simulink model "ME655_Lect09_VL3_Simulink"  (R2023a)
settings: Solver=FixedStepAuto  StartTime=0.0  StopTime=60.0  FixedStep=.003  RelTol=1e-3
values from neighbouring files (symbols this model uses):
  A = [1 T; 0 1]    [MATLAB.m]    (also in ME655_Lect09_VL3_MATLAB.m)
  big_K = S_P * C / (S_H)    [MATLAB.m]    (also in ME655_Lect09_VL3_MATLAB.m)
  dt_active_control = 10    [MATLAB.m]    (also in ME655_Lect09_VL3_MATLAB.m)
  epsilon = 12    [MATLAB.m]    (also in ME655_Lect09_VL3_MATLAB.m)
  h = 2.5*N    (= 200)    [MATLAB.m]    (also in ME655_Lect09_VL3_MATLAB.m)
  lambda = .95    (= 0.95)    [MATLAB.m]    (also in ME655_Lect09_VL3_MATLAB.m)
  Lhip_pos0 = Lhip_pos(1)    [MATLAB.m]    (also in ME655_Lect09_VL3_MATLAB.m)
  Lhip_vel0 = Lhip_vel(1)    [MATLAB.m]    (also in ME655_Lect09_VL3_MATLAB.m)
  M = 6    [MATLAB.m]    (also in ME655_Lect09_VL3_MATLAB.m)
  N = 80    [MATLAB.m]    (also in ME655_Lect09_VL3_MATLAB.m)
  nu = .5    (= 0.5)    [MATLAB.m]    (also in ME655_Lect09_VL3_MATLAB.m)
  Q = G * G' * var(Lhip_a)    [MATLAB.m]    (also in ME655_Lect09_VL3_MATLAB.m)
  R = [var(phiP_dot_hat - Lhip_v) 0; 0 var(phiP_hat - Lhip_p)]    [MATLAB.m]    (also in ME655_Lect09_VL3_MATLAB.m)
  small_k = (-1) * big_K * phiH_avg' + phiP_avg'    [MATLAB.m]    (also in ME655_Lect09_VL3_MATLAB.m)
  t_start = 5.0    (= 5)    [MATLAB.m]    (also in ME655_Lect09_VL3_MATLAB.m)
  Tau_h_max = 30    [MATLAB.m]    (also in ME655_Lect09_VL3_MATLAB.m)
undefined symbols (not defined in the file or in its folder): Bh, g, IHC, IRC, Kh, LH, LR, mH, mR, theta_0, theta_d0
settings Model: Creator=Damiano  LastModifiedBy=hunte
settings SolverCC: AlgebraicLoopSolver=TrustRegion
settings DataIOCC: ReturnWorkspaceOutputs=off
settings DebuggingCC: UnconnectedInputMsg=warning  UnconnectedOutputMsg=warning  UnconnectedLineMsg=warning  ArithmeticOperatorsInVariantConditions=warning
settings ModelReferenceCC: EnableRefExpFcnMdlSchedulingChecks=on
settings SFSimCC: SimUseLocalCustomCode=off  CustomCodeUndefinedFunction=UseInterfaceOnly
settings RTWCC: RTWUseLocalCustomCode=off  DLArmComputeVersion=19.05
settings CodeAppCC: StateflowObjectComments=on

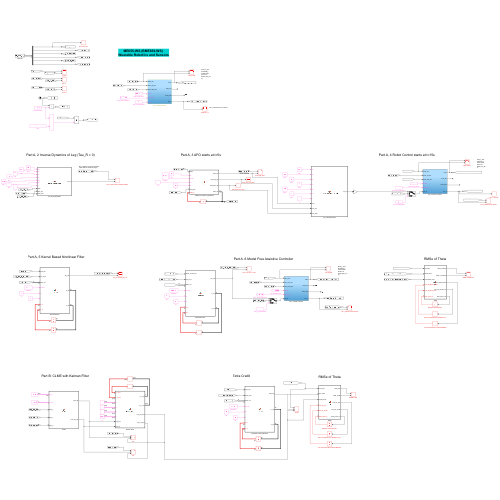
[thumbnail: Simulink's stored preview of the top-level diagram]
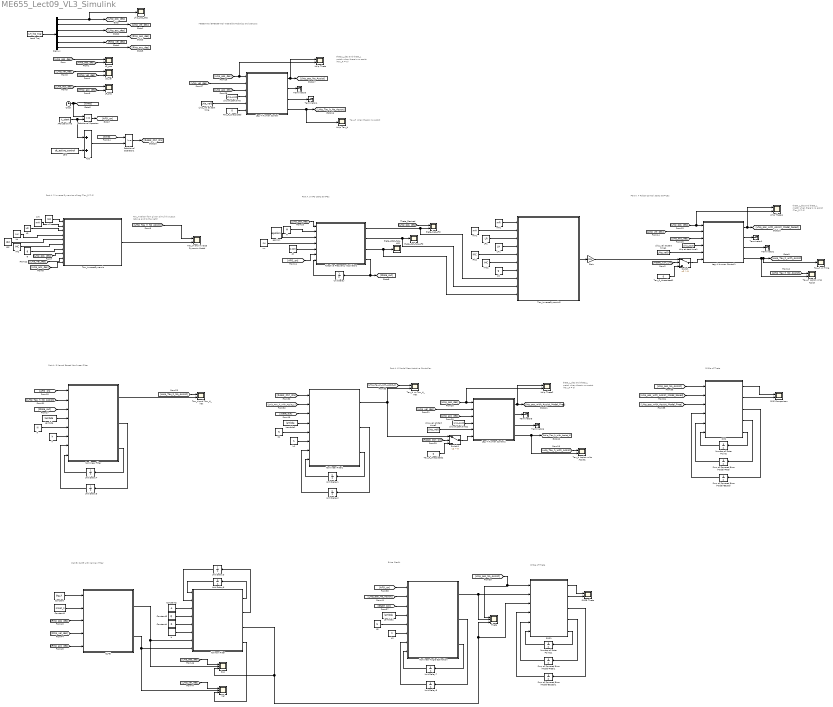
== system ME655_Lect09_VL3_Simulink ==
  note: Part A, 4 Robot Control starts at t=15s
  note: theta_L_des and theta_L match when there's no assist (Tau_R = 0)
  note: Part A, 5 Kernel Based Nonlinear Filter
  note: Part A, 3 AFO starts at t=5s
  note: theta_L_des and theta_L match when there's no assist (Tau_R = 0)
  note: ME655-WS (BME656-WS)
      | Wearable Robotics and Sensors
  note: Tau_H taken from given Simulink output (above and to the right)
  note: Part A, 2 Inverse Dynamics of Leg (Tau_R = 0)
  note: Tau_H when there's no assist
  note: theta_L_des and theta_L match when there's no assist (Tau_R = 0)
  note: Part A, 6 Model Free Assistive Controller
  note: RMSe of Theta
  note: Part B: CLME with Kalman Filter
  note: Extra Credit
  note: RMSe of Theta
  AFO start time : Constant  Value=t_start
  Adaptive Frequency Oscillators : MATLAB Function  TreatAsAtomicUnit=on
  Add : Sum
  CLME : MATLAB Function  TreatAsAtomicUnit=on
  Clock : Clock
  Constant : Constant  Value=big_K
  Constant1 : Constant  Value=small_k
  Constant2 : Constant  Value=A
  Constant3 : Constant  Value=Q
  Constant4 : Constant  Value=R
  Demux : Demux  Outputs=6
  Gain : Gain  Gain=0.5
  H : Constant  Value=eye(2)
  IHC : Constant  Value=IHC
  IHC1 : Constant  Value=IHC
  IRC : Constant  Value=IRC
  IRC1 : Constant  Value=IRC
  Kalman Filter : MATLAB Function  TreatAsAtomicUnit=on
  LH : Constant  Value=LH
  LH1 : Constant  Value=LH
  LHip Tau_H : Scope
  LHip Theta : Scope  NumInputPorts=2
  LHip Theta1 : Scope  NumInputPorts=2
  LHip Theta2 : Scope  NumInputPorts=2
  LR : Constant  Value=LR
  LR1 : Constant  Value=LR
  "LR_acc " : Scope  NumInputPorts=2
  LR_pos : Scope  NumInputPorts=2
  LR_vel : Scope  NumInputPorts=2
  Lambda : Constant  Value=lambda
  Lambda1 : Constant  Value=lambda
  Lambda2 : Constant  Value=lambda
  Leg + Human Control : Subsystem
  Leg + Human Control1 : Subsystem
  Leg + Human Control2 : Subsystem
  Lhip at start time : Constant  Value=Lhip_pos0
  Lhip at start time1 : Constant  Value=Lhip_pos0
  Lhip at start time2 : Constant  Value=Lhip_pos0
  Lhip_pos_des : Scope
  Lhip_vel at start time : Constant  Value=Lhip_vel0
  Lhip_vel at start time1 : Constant  Value=Lhip_vel0
  Lhip_vel at start time2 : Constant  Value=Lhip_vel0
  Load Traj : FromWorkspace  VariableName=LH_hip_traj
  M : Constant  Value=M
  N : Constant  Value=N
  N1 : Constant  Value=N
  N2 : Constant  Value=N
  Nonlinear Angle Estimation : MATLAB Function  TreatAsAtomicUnit=on
  Nonlinear Filter : MATLAB Function  TreatAsAtomicUnit=on
  Nonlinear Filter1 : MATLAB Function  TreatAsAtomicUnit=on
  Number of Data Points : UnitDelay  SampleTime=-1  HasFrameUpgradeWarning=on
  Number of Data Points1 : UnitDelay  SampleTime=-1  HasFrameUpgradeWarning=on
  Pos : Scope  NumInputPorts=3
  RMS : MATLAB Function  TreatAsAtomicUnit=on
  RMS Comparison : Scope  NumInputPorts=2
  RMS1 : MATLAB Function  TreatAsAtomicUnit=on
  RMSE Theta : Scope  NumInputPorts=2
  Relational Operator : RelationalOperator  OutDataTypeStr=boolean  RndMeth=Simplest  InputSameDT=off
  Relational Operator1 : RelationalOperator  OutDataTypeStr=boolean  RndMeth=Simplest  InputSameDT=off
  Sum of Squared Error (Model-Based) : UnitDelay  SampleTime=-1  HasFrameUpgradeWarning=on
  Sum of Squared Error (Model-Based)1 : UnitDelay  SampleTime=-1  HasFrameUpgradeWarning=on
  Sum of Squared Error (Model-Free) : UnitDelay  SampleTime=-1  HasFrameUpgradeWarning=on
  Sum of Squared Error (Model-Free)1 : UnitDelay  SampleTime=-1  HasFrameUpgradeWarning=on
  Switch : Switch  Criteria=u2 > Threshold  SaturateOnIntegerOverflow=off  InputSameDT=off
  Switch1 : Switch  Criteria=u2 > Threshold  SaturateOnIntegerOverflow=off  InputSameDT=off
  Tau_H Assist vs No Assist : Scope  NumInputPorts=2
  Tau_H Assist vs No Assist1 : Scope  NumInputPorts=2
  Tau_H and Inverse Dynamic Model : Scope  NumInputPorts=2
  Tau_H and Tau_H_hat : Scope  NumInputPorts=2
  Tau_H vs Tau_H_Hat : Scope  NumInputPorts=2
  Tau_InverseDynamic : MATLAB Function  TreatAsAtomicUnit=on
  Tau_InverseDynamic2 : MATLAB Function  TreatAsAtomicUnit=on
  Tau_R_Unassisted : Constant  Value=0
  Tau_R_Unassisted1 : Constant  Value=0
  Tau_R_Unassisted2 : Constant  Value=0
  Tau_h vs Time : Scope
  Terminator{1..6} (6 alike) : Terminator
  Theta : Scope  NumInputPorts=3
  Unit Delay : UnitDelay  InitialCondition=[0; 3*pi/2; pi/2; pi/2; pi/2; pi/2; pi/2; pi/2; 0; 0; 0; 0; 0; 0];  SampleTime=-1  HasFrameUpgradeWarning=on
  Unit Delay1 : UnitDelay  InitialCondition=zeros([N,1])  SampleTime=-1  HasFrameUpgradeWarning=on
  Unit Delay2 : UnitDelay  InitialCondition=ones([N,1])  SampleTime=-1  HasFrameUpgradeWarning=on
  Unit Delay3 : UnitDelay  InitialCondition=eye(2)  SampleTime=-1  HasFrameUpgradeWarning=on
  Unit Delay4 : UnitDelay  InitialCondition=zeros([N,1])  SampleTime=-1  HasFrameUpgradeWarning=on
  Unit Delay5 : UnitDelay  InitialCondition=ones([N,1])  SampleTime=-1  HasFrameUpgradeWarning=on
  Unit Delay6 : UnitDelay  InitialCondition=[0;0]  SampleTime=-1  HasFrameUpgradeWarning=on
  Unit Delay7 : UnitDelay  InitialCondition=zeros([N,1])  SampleTime=-1  HasFrameUpgradeWarning=on
  Unit Delay8 : UnitDelay  InitialCondition=ones([N,1])  SampleTime=-1  HasFrameUpgradeWarning=on
  Vel : Scope  NumInputPorts=3
  dt : Constant  Value=0.003
  epsilon : Constant  Value=epsilon
  g : Constant  Value=g
  g1 : Constant  Value=g
  h : Constant  Value=h
  h1 : Constant  Value=h
  h2 : Constant  Value=h
  mH : Constant  Value=mH
  mH1 : Constant  Value=mH
  mR : Constant  Value=mR
  mR1 : Constant  Value=mR
  nu : Constant  Value=nu
  theta_ddot_hat_AFO : Scope
  theta_dot_hat_AFO : Scope
  theta_hat_AFO : Scope  NumInputPorts=2
  zero : Constant  Value=dt_active_control
  wires:
  Tau_InverseDynamic2/1(Tau_tot) -> Gain/1
  IHC1/1 -> Tau_InverseDynamic2/6(IHC)
  IRC1/1 -> Tau_InverseDynamic2/5(IRC)
  g1/1 -> Tau_InverseDynamic2/7(g)
  LH1/1 -> Tau_InverseDynamic2/4(LH)
  LR1/1 -> Tau_InverseDynamic2/3(LR)
  mH1/1 -> Tau_InverseDynamic2/2(mH)
  mR1/1 -> Tau_InverseDynamic2/1(mR)
  [Lhip_pos_des] -> LHip Theta1/2, Leg + Human Control1/1(theta_des)
  Leg + Human Control1/4(Tau_h) -> Tau_h vs Time/1, [LHip_Tau_h_with_Assist], Tau_H Assist vs No Assist/2
  Leg + Human Control1/1(theta) -> [Lhip_pos_with_Assist_Model_based], LHip Theta1/1
  Lhip at start time1/1 -> Leg + Human Control1/4(theta0)
  [Lhip_vel_des] -> Leg + Human Control1/2(theta_dot_des)
  Leg + Human Control1/2(theta_dot) -> Terminator1/1
  Lhip_vel at start time1/1 -> Leg + Human Control1/5(theta0_dot)
  Leg + Human Control1/3(theta_ddot) -> Terminator2/1
  [Lhip_acc_des] -> Leg + Human Control1/3(theta_ddot_des)
  Gain/1 -> Switch/1
  Unit Delay4/1 -> Nonlinear Filter/8(w_in)
  h/1 -> Nonlinear Filter/6(h)
  Lambda/1 -> Nonlinear Filter/4(lambda)
  Nonlinear Filter/3(w_out) -> Unit Delay4/1
  Unit Delay5/1 -> Nonlinear Filter/7(P_in)
  N/1 -> Nonlinear Filter/5(N)
  [LHip_Tau_h_No_Assist] -> Nonlinear Filter/2(Tau_input)
  [State_out] -> Nonlinear Filter/3(State_out)
  LH/1 -> Tau_InverseDynamic/4(LH)
  Demux/2 -> [Lhip_vel_des]
  [Lhip_pos_des] -> theta_hat_AFO/1
  epsilon/1 -> Adaptive Frequency Oscillators/3(epsilon)
  Lhip at start time/1 -> Leg + Human Control/4(theta0)
  Demux/1 -> Lhip_pos_des/1, [Lhip_pos_des]
  Demux/6 -> [Rhip_acc_des]
  nu/1 -> Adaptive Frequency Oscillators/4(nu)
  Leg + Human Control/1(theta) -> LHip Theta/1, [Lhip_pos_No_Assist]
  Relational Operator/1 -> [AFO_on]
  LR/1 -> Tau_InverseDynamic/3(LR)
  [AFO_on] -> Adaptive Frequency Oscillators/6(AFO_ON)
  Adaptive Frequency Oscillators/3(theta_ddot_hat) -> Tau_InverseDynamic2/10(theta_ddot), theta_ddot_hat_AFO/1
  M/1 -> Adaptive Frequency Oscillators/2(M)
  Unit Delay/1 -> Adaptive Frequency Oscillators/7(state_in)
  Tau_InverseDynamic/1(Tau_tot) -> Tau_H and Inverse Dynamic Model/2
  Adaptive Frequency Oscillators/4(state_out) -> Unit Delay/1, [State_out]
  Demux/3 -> [Lhip_acc_des]
  Relational Operator1/1 -> [Robot_Ctrl_ON]
  [Lhip_acc_des] -> Tau_InverseDynamic/10(theta_ddot)
  [Lhip_acc_des] -> "LR_acc "/1
  Adaptive Frequency Oscillators/2(theta_dot_hat) -> Tau_InverseDynamic2/9(theta_dot), theta_dot_hat_AFO/1
  Leg + Human Control/2(theta_dot) -> Terminator3/1
  mH/1 -> Tau_InverseDynamic/2(mH)
  [Lhip_vel_des] -> LR_vel/1
  IHC/1 -> Tau_InverseDynamic/6(IHC)
  Leg + Human Control/4(Tau_h) -> LHip Tau_H/1, [LHip_Tau_h_No_Assist]
  g/1 -> Tau_InverseDynamic/7(g)
  Tau_R_Unassisted/1 -> Leg + Human Control/6(Tau_R)
  Adaptive Frequency Oscillators/1(theta_hat) -> Tau_InverseDynamic2/8(theta), theta_hat_AFO/2
  [Lhip_pos_des] -> Tau_InverseDynamic/8(theta)
  [LHip_Tau_h_No_Assist] -> Tau_H and Inverse Dynamic Model/1
  dt/1 -> Adaptive Frequency Oscillators/5(dt)
  zero/1 -> Add/2
  mR/1 -> Tau_InverseDynamic/1(mR)
  [Lhip_pos_des] -> Leg + Human Control/1(theta_des), LHip Theta/2
  [Lhip_acc_des] -> Leg + Human Control/3(theta_ddot_des)
  [Lhip_vel_des] -> Tau_InverseDynamic/9(theta_dot)
  [Lhip_pos_des] -> LR_pos/1
  Add/1 -> Relational Operator1/2
  IRC/1 -> Tau_InverseDynamic/5(IRC)
  [Rhip_vel_des] -> LR_vel/2
  Clock/1 -> Relational Operator/1, [time]
  Load Traj/1 -> Demux/1
  [Rhip_acc_des] -> "LR_acc "/2
  [Lhip_pos_des] -> Adaptive Frequency Oscillators/1(theta)
  [Lhip_vel_des] -> Leg + Human Control/2(theta_dot_des)
  Leg + Human Control/3(theta_ddot) -> Terminator4/1
  [time] -> Relational Operator1/1
  AFO start time/1 -> Add/1, Relational Operator/2
  Demux/4 -> [Rhip_pos_des]
  Demux/5 -> [Rhip_vel_des]
  Lhip_vel at start time/1 -> Leg + Human Control/5(theta0_dot)
  [Rhip_pos_des] -> LR_pos/2
  [LHip_Tau_h_No_Assist] -> Tau_H Assist vs No Assist/1
  Tau_R_Unassisted1/1 -> Switch/3
  [Robot_Ctrl_ON] -> Switch/2
  Switch/1 -> Leg + Human Control1/6(Tau_R)
  [AFO_on] -> Nonlinear Filter/1(AFO_ON)
  [LHip_Tau_h_No_Assist] -> Tau_H and Tau_H_hat/1
  [Robot_Ctrl_ON] -> Switch1/2
  Switch1/1 -> Leg + Human Control2/6(Tau_R)
  Nonlinear Filter/2(P_out) -> Unit Delay5/1
  Tau_R_Unassisted2/1 -> Switch1/3
  Lhip_vel at start time2/1 -> Leg + Human Control2/5(theta0_dot)
  [Lhip_pos_des] -> LHip Theta2/2, Leg + Human Control2/1(theta_des)
  Leg + Human Control2/3(theta_ddot) -> Terminator6/1
  Leg + Human Control2/1(theta) -> [Lhip_pos_with_Assist_Model_Free], LHip Theta2/1
  [Lhip_vel_des] -> Leg + Human Control2/2(theta_dot_des)
  Leg + Human Control2/4(Tau_h) -> [LHip_Tau_h_with_Assist_1], Tau_H Assist vs No Assist1/2
  [Lhip_acc_des] -> Leg + Human Control2/3(theta_ddot_des)
  Lhip at start time2/1 -> Leg + Human Control2/4(theta0)
  [LHip_Tau_h_with_Assist] -> Tau_H Assist vs No Assist1/1
  Leg + Human Control2/2(theta_dot) -> Terminator5/1
  Nonlinear Filter/1(Tau_hat) -> Tau_H and Tau_H_hat/2
  Nonlinear Filter1/2(P_out) -> Unit Delay2/1
  [Robot_Ctrl_ON] -> Nonlinear Filter1/1(Robot_Control_ON)
  [State_out] -> Nonlinear Filter1/3(State_out)
  [LHip_Tau_h_with_Assist_1] -> Nonlinear Filter1/2(Tau_input)
  N1/1 -> Nonlinear Filter1/5(N)
  Unit Delay2/1 -> Nonlinear Filter1/7(P_in)
  Nonlinear Filter1/3(w_out) -> Unit Delay1/1
  Lambda1/1 -> Nonlinear Filter1/4(lambda)
  h1/1 -> Nonlinear Filter1/6(h)
  Unit Delay1/1 -> Nonlinear Filter1/8(w_in)
  Nonlinear Filter1/1(Tau_hat) -> Tau_H vs Tau_H_Hat/2, Switch1/1
  [LHip_Tau_h_with_Assist_1] -> Tau_H vs Tau_H_Hat/1
  [Lhip_pos_with_Assist_Model_Free] -> RMS/3(Unmodeled_theta)
  [Lhip_pos_No_Assist] -> RMS/1(Act_theta)
  [Lhip_pos_with_Assist_Model_based] -> RMS/2(Model_theta)
  Number of Data Points/1 -> RMS/6(Data_points_in)
  Sum of Squared Error (Model-Free)/1 -> RMS/5("Sum_E2_Model_free ")
  Sum of Squared Error (Model-Based)/1 -> RMS/4("Sum_E2_Model_based ")
  RMS/1(RMS_modeled) -> RMS Comparison/1
  RMS/2(RMS_unmodeled) -> RMS Comparison/2
  RMS/5(Data_points_out) -> Number of Data Points/1
  RMS/4(Sum_E2_Model_free) -> Sum of Squared Error (Model-Free)/1
  RMS/3(Sum_E2_Model_based) -> Sum of Squared Error (Model-Based)/1
  CLME/2(phiP_dot_hat) -> Kalman Filter/8(Lhip_vel), Vel/2
  Unit Delay3/1 -> Kalman Filter/2(P_k_prev)
  [Rhip_pos_des] -> CLME/3(Rhip_p)
  [Rhip_acc_des] -> CLME/5(Rhip_a)
  CLME/1(phiP_hat) -> Kalman Filter/7(Lhip_pos), Pos/2
  [Rhip_vel_des] -> CLME/4(Rhip_v)
  Kalman Filter/2(P_k_next) -> Unit Delay3/1
  Unit Delay6/1 -> Kalman Filter/1(x_k_prev)
  Kalman Filter/1(x_k_next) -> Unit Delay6/1
  H/1 -> Kalman Filter/6(H)
  Kalman Filter/4(Lhip_vel_des) -> Vel/3
  [Lhip_pos_des] -> Pos/1
  [Lhip_vel_des] -> Vel/1
  Constant1/1 -> CLME/2(small_k)
  Constant/1 -> CLME/1(big_K)
  Constant2/1 -> Kalman Filter/3(A)
  Constant3/1 -> Kalman Filter/4(Q)
  Constant4/1 -> Kalman Filter/5(R)
  N2/1 -> Nonlinear Angle Estimation/5(N)
  h2/1 -> Nonlinear Angle Estimation/6(h)
  Nonlinear Angle Estimation/2(P_out) -> Unit Delay8/1
  Nonlinear Angle Estimation/3(w_out) -> Unit Delay7/1
  Lambda2/1 -> Nonlinear Angle Estimation/4(lambda)
  Unit Delay8/1 -> Nonlinear Angle Estimation/7(P_in)
  [State_out] -> Nonlinear Angle Estimation/3(State_out)
  [AFO_on] -> Nonlinear Angle Estimation/1(AFO_ON)
  Unit Delay7/1 -> Nonlinear Angle Estimation/8(w_in)
  [Lhip_pos_No_Assist] -> Nonlinear Angle Estimation/2(theta_input)
  RMS1/3(Sum_E2_NLF) -> Sum of Squared Error (Model-Based)1/1
  RMS1/4(Sum_E2_CLME) -> Sum of Squared Error (Model-Free)1/1
  Sum of Squared Error (Model-Free)1/1 -> RMS1/5(Sum_E_CLME)
  RMS1/5(Data_points_out) -> Number of Data Points1/1
  Number of Data Points1/1 -> RMS1/6(Data_points_in)
  Kalman Filter/3(Lhip_pos_des) -> Pos/3, Theta/3, RMS1/3(CLME_theta)
  [Lhip_pos_No_Assist] -> Theta/1, RMS1/1(Act_theta)
  Nonlinear Angle Estimation/1(theta_hat) -> RMS1/2(NLF_theta), Theta/2
  Sum of Squared Error (Model-Based)1/1 -> RMS1/4(Sum_E_NLF)
  RMS1/1(RMS_NLF) -> RMSE Theta/1
  RMS1/2(RMS_CLME) -> RMSE Theta/2

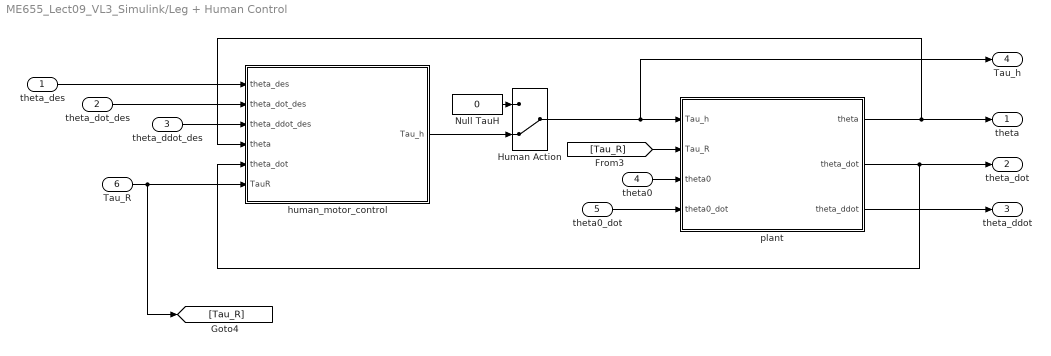
== system ME655_Lect09_VL3_Simulink/Leg + Human Control ==
  theta_des : Inport
  theta_dot_des : Inport  Port=2
  theta_ddot_des : Inport  Port=3
  theta0 : Inport  Port=4
  theta0_dot : Inport  Port=5
  Tau_R : Inport  Port=6
  Human Action : ManualSwitch  CurrentSetting=0
  Null TauH : Constant  Value=0
  human_motor_control : Subsystem
  plant : Subsystem
  theta : Outport  PortDimensions=[1,1]  VectorParamsAs1DForOutWhenUnconnected=off
  theta_dot : Outport  Port=2  PortDimensions=[1,1]  VectorParamsAs1DForOutWhenUnconnected=off
  theta_ddot : Outport  Port=3  PortDimensions=[1,1]  VectorParamsAs1DForOutWhenUnconnected=off
  Tau_h : Outport  Port=4  PortDimensions=[1,1]  VectorParamsAs1DForOutWhenUnconnected=off
  wires:
  theta_des/1 -> human_motor_control/1(theta_des)
  theta_dot_des/1 -> human_motor_control/2(theta_dot_des)
  theta0/1 -> plant/3(theta0)
  theta0_dot/1 -> plant/4(theta0_dot)
  [Tau_R] -> plant/2(Tau_R)
  plant/1(theta) -> theta/1, human_motor_control/4(theta)
  plant/2(theta_dot) -> human_motor_control/5(theta_dot), theta_dot/1
  plant/3(theta_ddot) -> theta_ddot/1
  theta_ddot_des/1 -> human_motor_control/3(theta_ddot_des)
  human_motor_control/1(Tau_h) -> Human Action/2
  Human Action/1 -> Tau_h/1, plant/1(Tau_h)
  Null TauH/1 -> Human Action/1
  Tau_R/1 -> [Tau_R], human_motor_control/6(TauR)

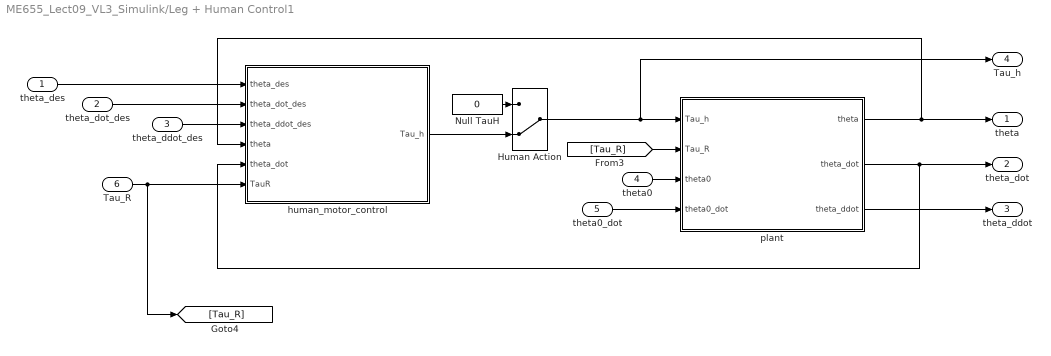
== system ME655_Lect09_VL3_Simulink/Leg + Human Control1 ==
  theta_des : Inport
  theta_dot_des : Inport  Port=2
  theta_ddot_des : Inport  Port=3
  theta0 : Inport  Port=4
  theta0_dot : Inport  Port=5
  Tau_R : Inport  Port=6
  Human Action : ManualSwitch  CurrentSetting=0
  Null TauH : Constant  Value=0
  human_motor_control : Subsystem
  plant : Subsystem
  theta : Outport  PortDimensions=[1,1]  VectorParamsAs1DForOutWhenUnconnected=off
  theta_dot : Outport  Port=2  PortDimensions=[1,1]  VectorParamsAs1DForOutWhenUnconnected=off
  theta_ddot : Outport  Port=3  PortDimensions=[1,1]  VectorParamsAs1DForOutWhenUnconnected=off
  Tau_h : Outport  Port=4  PortDimensions=[1,1]  VectorParamsAs1DForOutWhenUnconnected=off
  wires:
  Tau_R/1 -> human_motor_control/6(TauR), [Tau_R]
  Null TauH/1 -> Human Action/1
  Human Action/1 -> plant/1(Tau_h), Tau_h/1
  human_motor_control/1(Tau_h) -> Human Action/2
  theta_ddot_des/1 -> human_motor_control/3(theta_ddot_des)
  plant/3(theta_ddot) -> theta_ddot/1
  plant/2(theta_dot) -> theta_dot/1, human_motor_control/5(theta_dot)
  plant/1(theta) -> human_motor_control/4(theta), theta/1
  [Tau_R] -> plant/2(Tau_R)
  theta0_dot/1 -> plant/4(theta0_dot)
  theta0/1 -> plant/3(theta0)
  theta_dot_des/1 -> human_motor_control/2(theta_dot_des)
  theta_des/1 -> human_motor_control/1(theta_des)

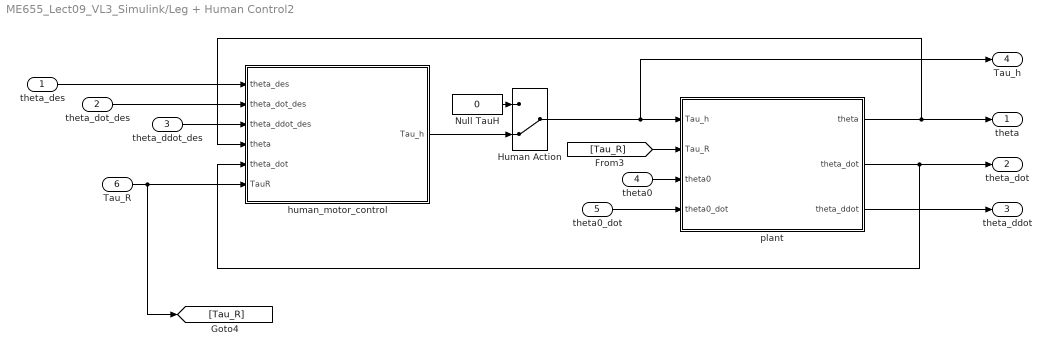
== system ME655_Lect09_VL3_Simulink/Leg + Human Control2 ==
  theta_des : Inport
  theta_dot_des : Inport  Port=2
  theta_ddot_des : Inport  Port=3
  theta0 : Inport  Port=4
  theta0_dot : Inport  Port=5
  Tau_R : Inport  Port=6
  Human Action : ManualSwitch  CurrentSetting=0
  Null TauH : Constant  Value=0
  human_motor_control : Subsystem
  plant : Subsystem
  theta : Outport  PortDimensions=[1,1]  VectorParamsAs1DForOutWhenUnconnected=off
  theta_dot : Outport  Port=2  PortDimensions=[1,1]  VectorParamsAs1DForOutWhenUnconnected=off
  theta_ddot : Outport  Port=3  PortDimensions=[1,1]  VectorParamsAs1DForOutWhenUnconnected=off
  Tau_h : Outport  Port=4  PortDimensions=[1,1]  VectorParamsAs1DForOutWhenUnconnected=off
  wires:
  Tau_R/1 -> human_motor_control/6(TauR), [Tau_R]
  Null TauH/1 -> Human Action/1
  Human Action/1 -> plant/1(Tau_h), Tau_h/1
  human_motor_control/1(Tau_h) -> Human Action/2
  theta_ddot_des/1 -> human_motor_control/3(theta_ddot_des)
  plant/3(theta_ddot) -> theta_ddot/1
  plant/2(theta_dot) -> theta_dot/1, human_motor_control/5(theta_dot)
  plant/1(theta) -> human_motor_control/4(theta), theta/1
  [Tau_R] -> plant/2(Tau_R)
  theta0_dot/1 -> plant/4(theta0_dot)
  theta0/1 -> plant/3(theta0)
  theta_dot_des/1 -> human_motor_control/2(theta_dot_des)
  theta_des/1 -> human_motor_control/1(theta_des)

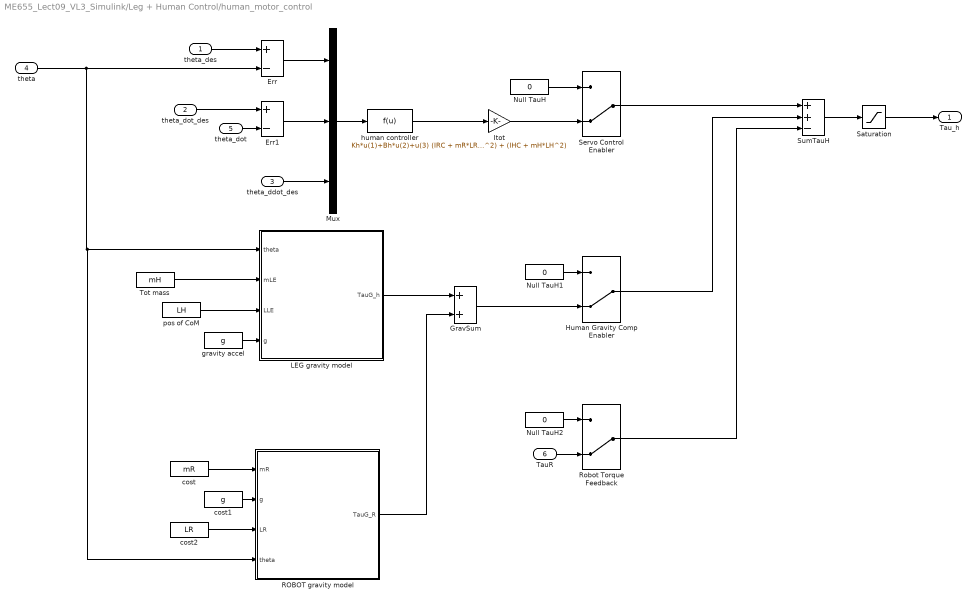
== system ME655_Lect09_VL3_Simulink/Leg + Human Control/human_motor_control ==
  theta_des : Inport
  theta_dot_des : Inport  Port=2
  theta_ddot_des : Inport  Port=3
  theta : Inport  Port=4
  theta_dot : Inport  Port=5
  TauR : Inport  Port=6
  Err : Sum  Inputs=+-
  Err1 : Sum  Inputs=+-
  GravSum : Sum
  Human Gravity Comp Enabler : ManualSwitch  CurrentSetting=0
  Itot : Gain  Gain=(IRC + mR*LR^2) + (IHC + mH*LH^2)
  LEG gravity model : MATLAB Function  TreatAsAtomicUnit=on
  Mux : Mux  Inputs=3
  Null TauH : Constant  Value=0
  Null TauH1 : Constant  Value=0
  Null TauH2 : Constant  Value=0
  ROBOT gravity model : MATLAB Function  TreatAsAtomicUnit=on
  Robot Torque Feedback : ManualSwitch  CurrentSetting=0
  Saturation : Saturate  UpperLimit=Tau_h_max  LowerLimit=-Tau_h_max
  Servo Control Enabler : ManualSwitch  CurrentSetting=0
  SumTauH : Sum  Inputs=++-
  Tot mass : Constant  Value=mH
  cost : Constant  Value=mR
  cost1 : Constant  Value=g
  cost2 : Constant  Value=LR
  gravity accel : Constant  Value=g
  human controller : Fcn  Expr=Kh*u(1)+Bh*u(2)+u(3)
  pos of CoM : Constant  Value=LH
  Tau_h : Outport  PortDimensions=[1,1]  VectorParamsAs1DForOutWhenUnconnected=off
  wires:
  theta_des/1 -> Err/1
  theta_dot_des/1 -> Err1/1
  theta_dot/1 -> Err1/2
  Err/1 -> Mux/1
  Err1/1 -> Mux/2
  Mux/1 -> human controller/1
  theta_ddot_des/1 -> Mux/3
  gravity accel/1 -> LEG gravity model/4(g)
  Tot mass/1 -> LEG gravity model/2(mLE)
  pos of CoM/1 -> LEG gravity model/3(LLE)
  Null TauH/1 -> Servo Control Enabler/1
  Null TauH1/1 -> Human Gravity Comp Enabler/1
  Human Gravity Comp Enabler/1 -> SumTauH/2
  SumTauH/1 -> Saturation/1
  human controller/1 -> Itot/1
  Servo Control Enabler/1 -> SumTauH/1
  Saturation/1 -> Tau_h/1
  Itot/1 -> Servo Control Enabler/2
  Null TauH2/1 -> Robot Torque Feedback/1
  TauR/1 -> Robot Torque Feedback/2
  Robot Torque Feedback/1 -> SumTauH/3
  theta/1 -> ROBOT gravity model/4(theta), LEG gravity model/1(theta), Err/2
  ROBOT gravity model/1(TauG_R) -> GravSum/2
  cost2/1 -> ROBOT gravity model/3(LR)
  cost/1 -> ROBOT gravity model/1(mR)
  cost1/1 -> ROBOT gravity model/2(g)
  LEG gravity model/1(TauG_h) -> GravSum/1
  GravSum/1 -> Human Gravity Comp Enabler/2

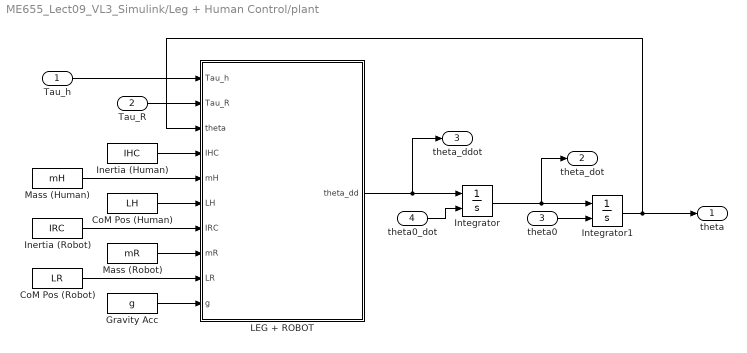
== system ME655_Lect09_VL3_Simulink/Leg + Human Control/plant ==
  Tau_h : Inport
  Tau_R : Inport  Port=2
  theta0 : Inport  Port=3
  theta0_dot : Inport  Port=4
  CoM Pos (Human) : Constant  Value=LH
  CoM Pos (Robot) : Constant  Value=LR
  Gravity Acc : Constant  Value=g
  Inertia (Human) : Constant  Value=IHC
  Inertia (Robot) : Constant  Value=IRC
  Integrator : Integrator  InitialConditionSource=external  InitialCondition=theta_d0
  Integrator1 : Integrator  InitialConditionSource=external  InitialCondition=theta_0
  LEG + ROBOT : MATLAB Function  TreatAsAtomicUnit=on
  Mass (Human) : Constant  Value=mH
  Mass (Robot) : Constant  Value=mR
  theta : Outport  PortDimensions=[1,1]  VectorParamsAs1DForOutWhenUnconnected=off
  theta_dot : Outport  Port=2  PortDimensions=[1,1]  VectorParamsAs1DForOutWhenUnconnected=off
  theta_ddot : Outport  Port=3  PortDimensions=[1,1]  VectorParamsAs1DForOutWhenUnconnected=off
  wires:
  Tau_h/1 -> LEG + ROBOT/1(Tau_h)
  Tau_R/1 -> LEG + ROBOT/2(Tau_R)
  LEG + ROBOT/1(theta_dd) -> theta_ddot/1, Integrator/1
  Integrator/1 -> theta_dot/1, Integrator1/1
  theta0_dot/1 -> Integrator/2
  theta0/1 -> Integrator1/2
  Integrator1/1 -> LEG + ROBOT/3(theta), theta/1
  Inertia (Human)/1 -> LEG + ROBOT/4(IHC)
  Mass (Human)/1 -> LEG + ROBOT/5(mH)
  CoM Pos (Human)/1 -> LEG + ROBOT/6(LH)
  Gravity Acc/1 -> LEG + ROBOT/10(g)
  Mass (Robot)/1 -> LEG + ROBOT/8(mR)
  CoM Pos (Robot)/1 -> LEG + ROBOT/9(LR)
  Inertia (Robot)/1 -> LEG + ROBOT/7(IRC)

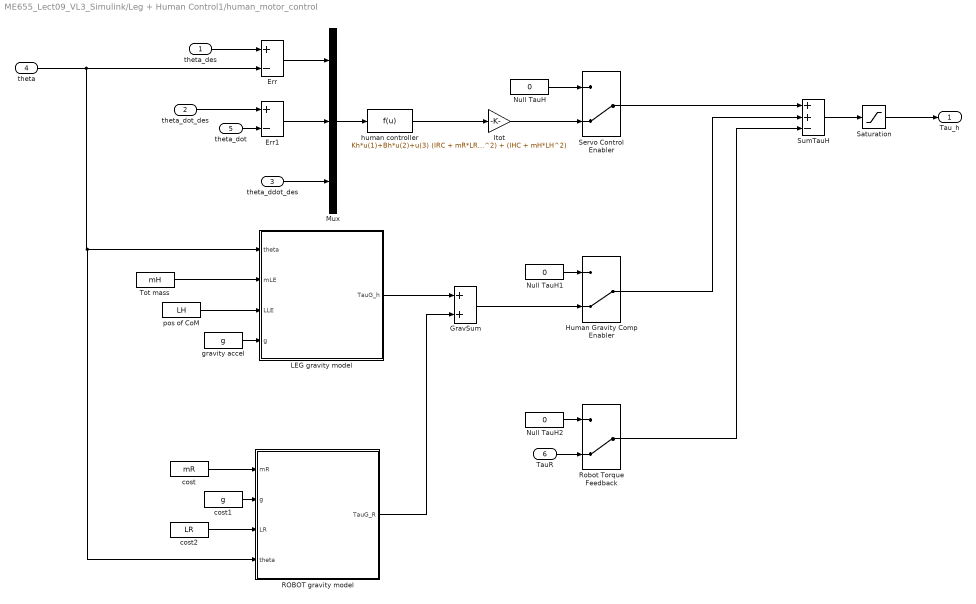
== system ME655_Lect09_VL3_Simulink/Leg + Human Control1/human_motor_control ==
  theta_des : Inport
  theta_dot_des : Inport  Port=2
  theta_ddot_des : Inport  Port=3
  theta : Inport  Port=4
  theta_dot : Inport  Port=5
  TauR : Inport  Port=6
  Err : Sum  Inputs=+-
  Err1 : Sum  Inputs=+-
  GravSum : Sum
  Human Gravity Comp Enabler : ManualSwitch  CurrentSetting=0
  Itot : Gain  Gain=(IRC + mR*LR^2) + (IHC + mH*LH^2)
  LEG gravity model : MATLAB Function  TreatAsAtomicUnit=on
  Mux : Mux  Inputs=3
  Null TauH : Constant  Value=0
  Null TauH1 : Constant  Value=0
  Null TauH2 : Constant  Value=0
  ROBOT gravity model : MATLAB Function  TreatAsAtomicUnit=on
  Robot Torque Feedback : ManualSwitch  CurrentSetting=0
  Saturation : Saturate  UpperLimit=Tau_h_max  LowerLimit=-Tau_h_max
  Servo Control Enabler : ManualSwitch  CurrentSetting=0
  SumTauH : Sum  Inputs=++-
  Tot mass : Constant  Value=mH
  cost : Constant  Value=mR
  cost1 : Constant  Value=g
  cost2 : Constant  Value=LR
  gravity accel : Constant  Value=g
  human controller : Fcn  Expr=Kh*u(1)+Bh*u(2)+u(3)
  pos of CoM : Constant  Value=LH
  Tau_h : Outport  PortDimensions=[1,1]  VectorParamsAs1DForOutWhenUnconnected=off
  wires:
  GravSum/1 -> Human Gravity Comp Enabler/2
  LEG gravity model/1(TauG_h) -> GravSum/1
  cost1/1 -> ROBOT gravity model/2(g)
  cost/1 -> ROBOT gravity model/1(mR)
  cost2/1 -> ROBOT gravity model/3(LR)
  ROBOT gravity model/1(TauG_R) -> GravSum/2
  theta/1 -> Err/2, LEG gravity model/1(theta), ROBOT gravity model/4(theta)
  Robot Torque Feedback/1 -> SumTauH/3
  TauR/1 -> Robot Torque Feedback/2
  Null TauH2/1 -> Robot Torque Feedback/1
  Itot/1 -> Servo Control Enabler/2
  Saturation/1 -> Tau_h/1
  Servo Control Enabler/1 -> SumTauH/1
  human controller/1 -> Itot/1
  SumTauH/1 -> Saturation/1
  Human Gravity Comp Enabler/1 -> SumTauH/2
  Null TauH1/1 -> Human Gravity Comp Enabler/1
  Null TauH/1 -> Servo Control Enabler/1
  pos of CoM/1 -> LEG gravity model/3(LLE)
  Tot mass/1 -> LEG gravity model/2(mLE)
  gravity accel/1 -> LEG gravity model/4(g)
  theta_ddot_des/1 -> Mux/3
  Mux/1 -> human controller/1
  Err1/1 -> Mux/2
  Err/1 -> Mux/1
  theta_dot/1 -> Err1/2
  theta_dot_des/1 -> Err1/1
  theta_des/1 -> Err/1

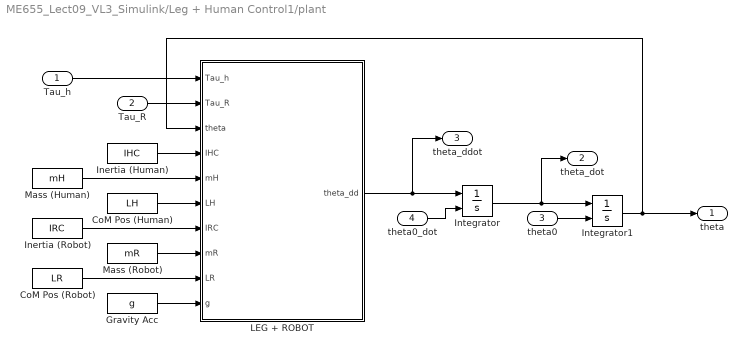
== system ME655_Lect09_VL3_Simulink/Leg + Human Control1/plant ==
  Tau_h : Inport
  Tau_R : Inport  Port=2
  theta0 : Inport  Port=3
  theta0_dot : Inport  Port=4
  CoM Pos (Human) : Constant  Value=LH
  CoM Pos (Robot) : Constant  Value=LR
  Gravity Acc : Constant  Value=g
  Inertia (Human) : Constant  Value=IHC
  Inertia (Robot) : Constant  Value=IRC
  Integrator : Integrator  InitialConditionSource=external  InitialCondition=theta_d0
  Integrator1 : Integrator  InitialConditionSource=external  InitialCondition=theta_0
  LEG + ROBOT : MATLAB Function  TreatAsAtomicUnit=on
  Mass (Human) : Constant  Value=mH
  Mass (Robot) : Constant  Value=mR
  theta : Outport  PortDimensions=[1,1]  VectorParamsAs1DForOutWhenUnconnected=off
  theta_dot : Outport  Port=2  PortDimensions=[1,1]  VectorParamsAs1DForOutWhenUnconnected=off
  theta_ddot : Outport  Port=3  PortDimensions=[1,1]  VectorParamsAs1DForOutWhenUnconnected=off
  wires:
  Inertia (Robot)/1 -> LEG + ROBOT/7(IRC)
  CoM Pos (Robot)/1 -> LEG + ROBOT/9(LR)
  Mass (Robot)/1 -> LEG + ROBOT/8(mR)
  Gravity Acc/1 -> LEG + ROBOT/10(g)
  CoM Pos (Human)/1 -> LEG + ROBOT/6(LH)
  Mass (Human)/1 -> LEG + ROBOT/5(mH)
  Inertia (Human)/1 -> LEG + ROBOT/4(IHC)
  Integrator1/1 -> theta/1, LEG + ROBOT/3(theta)
  theta0/1 -> Integrator1/2
  theta0_dot/1 -> Integrator/2
  Integrator/1 -> Integrator1/1, theta_dot/1
  LEG + ROBOT/1(theta_dd) -> Integrator/1, theta_ddot/1
  Tau_R/1 -> LEG + ROBOT/2(Tau_R)
  Tau_h/1 -> LEG + ROBOT/1(Tau_h)

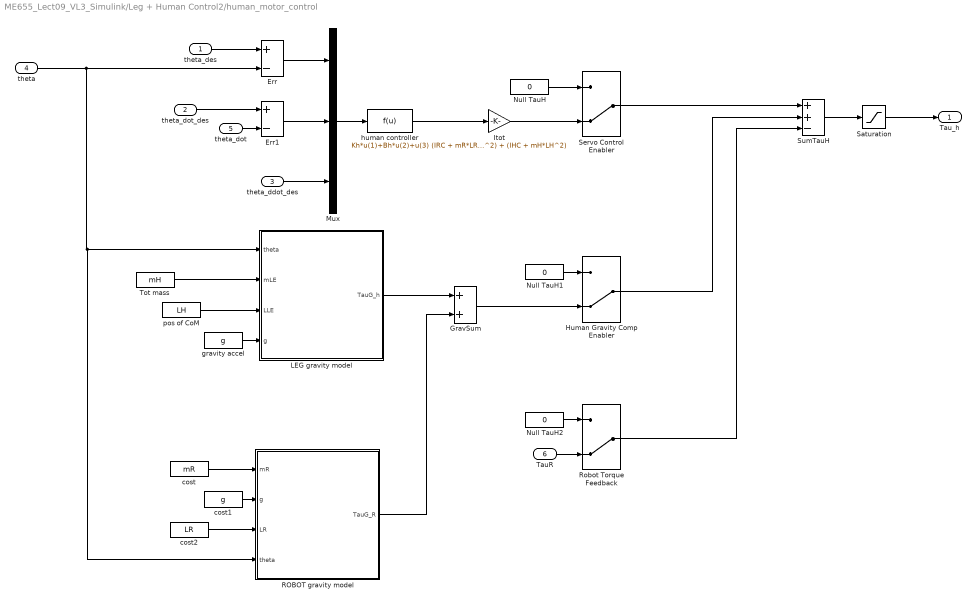
== system ME655_Lect09_VL3_Simulink/Leg + Human Control2/human_motor_control ==
  theta_des : Inport
  theta_dot_des : Inport  Port=2
  theta_ddot_des : Inport  Port=3
  theta : Inport  Port=4
  theta_dot : Inport  Port=5
  TauR : Inport  Port=6
  Err : Sum  Inputs=+-
  Err1 : Sum  Inputs=+-
  GravSum : Sum
  Human Gravity Comp Enabler : ManualSwitch  CurrentSetting=0
  Itot : Gain  Gain=(IRC + mR*LR^2) + (IHC + mH*LH^2)
  LEG gravity model : MATLAB Function  TreatAsAtomicUnit=on
  Mux : Mux  Inputs=3
  Null TauH : Constant  Value=0
  Null TauH1 : Constant  Value=0
  Null TauH2 : Constant  Value=0
  ROBOT gravity model : MATLAB Function  TreatAsAtomicUnit=on
  Robot Torque Feedback : ManualSwitch  CurrentSetting=0
  Saturation : Saturate  UpperLimit=Tau_h_max  LowerLimit=-Tau_h_max
  Servo Control Enabler : ManualSwitch  CurrentSetting=0
  SumTauH : Sum  Inputs=++-
  Tot mass : Constant  Value=mH
  cost : Constant  Value=mR
  cost1 : Constant  Value=g
  cost2 : Constant  Value=LR
  gravity accel : Constant  Value=g
  human controller : Fcn  Expr=Kh*u(1)+Bh*u(2)+u(3)
  pos of CoM : Constant  Value=LH
  Tau_h : Outport  PortDimensions=[1,1]  VectorParamsAs1DForOutWhenUnconnected=off
  wires:
  GravSum/1 -> Human Gravity Comp Enabler/2
  LEG gravity model/1(TauG_h) -> GravSum/1
  cost1/1 -> ROBOT gravity model/2(g)
  cost/1 -> ROBOT gravity model/1(mR)
  cost2/1 -> ROBOT gravity model/3(LR)
  ROBOT gravity model/1(TauG_R) -> GravSum/2
  theta/1 -> Err/2, LEG gravity model/1(theta), ROBOT gravity model/4(theta)
  Robot Torque Feedback/1 -> SumTauH/3
  TauR/1 -> Robot Torque Feedback/2
  Null TauH2/1 -> Robot Torque Feedback/1
  Itot/1 -> Servo Control Enabler/2
  Saturation/1 -> Tau_h/1
  Servo Control Enabler/1 -> SumTauH/1
  human controller/1 -> Itot/1
  SumTauH/1 -> Saturation/1
  Human Gravity Comp Enabler/1 -> SumTauH/2
  Null TauH1/1 -> Human Gravity Comp Enabler/1
  Null TauH/1 -> Servo Control Enabler/1
  pos of CoM/1 -> LEG gravity model/3(LLE)
  Tot mass/1 -> LEG gravity model/2(mLE)
  gravity accel/1 -> LEG gravity model/4(g)
  theta_ddot_des/1 -> Mux/3
  Mux/1 -> human controller/1
  Err1/1 -> Mux/2
  Err/1 -> Mux/1
  theta_dot/1 -> Err1/2
  theta_dot_des/1 -> Err1/1
  theta_des/1 -> Err/1

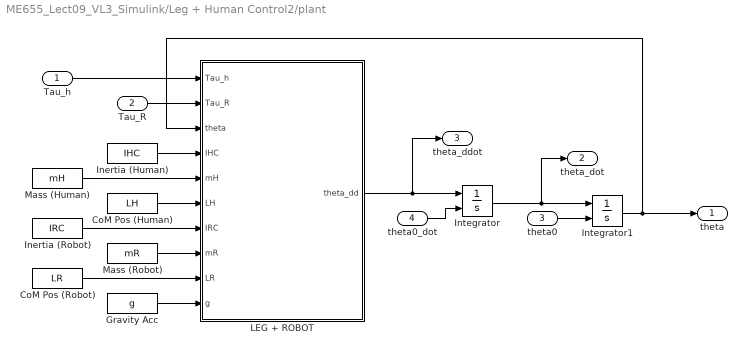
== system ME655_Lect09_VL3_Simulink/Leg + Human Control2/plant ==
  Tau_h : Inport
  Tau_R : Inport  Port=2
  theta0 : Inport  Port=3
  theta0_dot : Inport  Port=4
  CoM Pos (Human) : Constant  Value=LH
  CoM Pos (Robot) : Constant  Value=LR
  Gravity Acc : Constant  Value=g
  Inertia (Human) : Constant  Value=IHC
  Inertia (Robot) : Constant  Value=IRC
  Integrator : Integrator  InitialConditionSource=external  InitialCondition=theta_d0
  Integrator1 : Integrator  InitialConditionSource=external  InitialCondition=theta_0
  LEG + ROBOT : MATLAB Function  TreatAsAtomicUnit=on
  Mass (Human) : Constant  Value=mH
  Mass (Robot) : Constant  Value=mR
  theta : Outport  PortDimensions=[1,1]  VectorParamsAs1DForOutWhenUnconnected=off
  theta_dot : Outport  Port=2  PortDimensions=[1,1]  VectorParamsAs1DForOutWhenUnconnected=off
  theta_ddot : Outport  Port=3  PortDimensions=[1,1]  VectorParamsAs1DForOutWhenUnconnected=off
  wires:
  Inertia (Robot)/1 -> LEG + ROBOT/7(IRC)
  CoM Pos (Robot)/1 -> LEG + ROBOT/9(LR)
  Mass (Robot)/1 -> LEG + ROBOT/8(mR)
  Gravity Acc/1 -> LEG + ROBOT/10(g)
  CoM Pos (Human)/1 -> LEG + ROBOT/6(LH)
  Mass (Human)/1 -> LEG + ROBOT/5(mH)
  Inertia (Human)/1 -> LEG + ROBOT/4(IHC)
  Integrator1/1 -> theta/1, LEG + ROBOT/3(theta)
  theta0/1 -> Integrator1/2
  theta0_dot/1 -> Integrator/2
  Integrator/1 -> Integrator1/1, theta_dot/1
  LEG + ROBOT/1(theta_dd) -> Integrator/1, theta_ddot/1
  Tau_R/1 -> LEG + ROBOT/2(Tau_R)
  Tau_h/1 -> LEG + ROBOT/1(Tau_h)

== matlab function ME655_Lect09_VL3_Simulink/Nonlinear Filter ==
  data: AFO_ON input; Tau_hat output; Tau_input input; State_out input; lambda input; N input; h input; P_in input; w_in input; P_out output; w_out output
function [Tau_hat, P_out, w_out]= nonlin_filter(AFO_ON, Tau_input, State_out, lambda, N, h, P_in, w_in)

phi = State_out(3);

Tau_hat = 0;
P_out = P_in;
w_out = w_in;

if AFO_ON == 1

    Num = 0;
    Den = 0;
    err = zeros(N, 1);
    for i = 1:N
        psi = exp(h*(cos(phi - 2*pi*(i)/N)- 1));
        err(i) = Tau_input - w_in(i);
        P_out(i) = (1/lambda)*(P_in(i) - ((P_in(i)^2) / ((lambda/psi) + P_in(i))));    
        w_out(i) = w_in(i) + psi* P_out(i) * err(i);
        Num = Num + psi*w_in(i);
        Den = Den + psi;
    end

    Tau_hat = Num/Den;

end

== matlab function ME655_Lect09_VL3_Simulink/Leg + Human Control2/human_motor_control/LEG gravity model ==
  data: theta input; mLE input; LLE input; TauG_h output; g input
function TauG_h   = HumanLegGravModel(theta,mLE,LLE,g)
% human gravity compensation term
TauG_h=mLE*g*LLE*sin(theta);

end

== matlab function ME655_Lect09_VL3_Simulink/Leg + Human Control/human_motor_control/LEG gravity model ==
  data: theta input; mLE input; LLE input; TauG_h output; g input
function TauG_h   = HumanLegGravModel(theta,mLE,LLE,g)
% human gravity compensation term
TauG_h=mLE*g*LLE*sin(theta);

end

== matlab function ME655_Lect09_VL3_Simulink/Leg + Human Control2/human_motor_control/ROBOT gravity model ==
  data: mR input; g input; LR input; theta input; TauG_R output
function TauG_R  = RobotGravModel(mR,g,LR,theta)

TauG_R=mR*g*LR*sin(theta);
% TauG_h=mLE*g*LLE*sin(theta);

end

== matlab function ME655_Lect09_VL3_Simulink/Leg + Human Control2/plant/LEG + ROBOT ==
  data: Tau_h input; Tau_R input; theta input; theta_dd output; IHC input; mH input; LH input; IRC input; mR input; LR input; g input
function theta_dd   = LegRobotModel(Tau_h,Tau_R,theta,IHC,mH,LH,IRC,mR,LR,g)

theta_dd = 1/((IRC + mR*LR^2)+(IHC + mH*LH^2)) * (Tau_h-mH*g*LH*sin(theta) + Tau_R-mR*g*LR*sin(theta));

end

== matlab function ME655_Lect09_VL3_Simulink/Leg + Human Control/human_motor_control/ROBOT gravity model ==
  data: mR input; g input; LR input; theta input; TauG_R output
function TauG_R  = RobotGravModel(mR,g,LR,theta)

TauG_R=mR*g*LR*sin(theta);
% TauG_h=mLE*g*LLE*sin(theta);

end

== matlab function ME655_Lect09_VL3_Simulink/Nonlinear Filter1 ==
  data: Robot_Control_ON input; Tau_hat output; Tau_input input; State_out input; lambda input; N input; h input; P_in input; w_in input; P_out output; w_out output
function [Tau_hat, P_out, w_out]= nonlin_filter(Robot_Control_ON, Tau_input, State_out, lambda, N, h, P_in, w_in)

phi = State_out(3);

Tau_hat = 0;
P_out = P_in;
w_out = w_in;

if Robot_Control_ON == 1

    Num = 0;
    Den = 0;
    err = zeros(N, 1);
    for i = 1:N
        psi = exp(h*(cos(phi - 2*pi*(i)/N)- 1));
        err(i) = Tau_input - w_in(i);
        P_out(i) = (1/lambda)*(P_in(i) - ((P_in(i)^2) / ((lambda/psi) + P_in(i))));    
        w_out(i) = w_in(i) + psi* P_out(i) * err(i);
        Num = Num + psi*w_in(i);
        Den = Den + psi;
    end

    Tau_hat = Num/Den;

end

== matlab function ME655_Lect09_VL3_Simulink/Leg + Human Control/plant/LEG + ROBOT ==
  data: Tau_h input; Tau_R input; theta input; theta_dd output; IHC input; mH input; LH input; IRC input; mR input; LR input; g input
function theta_dd   = LegRobotModel(Tau_h,Tau_R,theta,IHC,mH,LH,IRC,mR,LR,g)

theta_dd = 1/((IRC + mR*LR^2)+(IHC + mH*LH^2)) * (Tau_h-mH*g*LH*sin(theta) + Tau_R-mR*g*LR*sin(theta));

end

== matlab function ME655_Lect09_VL3_Simulink/RMS ==
  data: Act_theta input; RMS_modeled output; RMS_unmodeled output; Sum_E2_Model_based output; Sum_E2_Model_free output; Data_points_out output; Model_theta input; Unmodeled_theta input; Sum_E2_Model_based input; Sum_E2_Model_free input; Data_points_in input
function [RMS_modeled, RMS_unmodeled, Sum_E2_Model_based, Sum_E2_Model_free, Data_points_out]= fcn(Act_theta, Model_theta, Unmodeled_theta, Sum_E2_Model_based, Sum_E2_Model_free, Data_points_in)

Data_points_out = Data_points_in + 1;
Sum_E2_Model_based = Sum_E2_Model_based + (Act_theta - Model_theta)^2;
Sum_E2_Model_free = Sum_E2_Model_free + (Act_theta - Unmodeled_theta)^2;
RMS_modeled= (Sum_E2_Model_based/Data_points_out)^(0.5);
RMS_unmodeled= (Sum_E2_Model_free/Data_points_out)^(0.5);

== matlab function ME655_Lect09_VL3_Simulink/Nonlinear Angle Estimation ==
  data: AFO_ON input; theta_hat output; theta_input input; State_out input; lambda input; N input; h input; P_in input; w_in input; P_out output; w_out output
function [theta_hat, P_out, w_out]= nonlin_filter(AFO_ON, theta_input, State_out, lambda, N, h, P_in, w_in)

% estimate theta_hat using psi-1
phi = State_out(3);

theta_hat = 0;
P_out = P_in;
w_out = w_in;

if AFO_ON == 1

    Num = 0;
    Den = 0;
    err = zeros(N, 1);
    for i = 1:N
        psi = phi;
        err(i) = theta_input - w_in(i);
        P_out(i) = (1/lambda)*(P_in(i) - ((P_in(i)^2) / ((lambda/psi) + P_in(i))));    
        w_out(i) = w_in(i) + psi* P_out(i) * err(i);
        Num = Num + psi*w_in(i);
        Den = Den + psi;
    end

    theta_hat = Num/Den;

end

== matlab function ME655_Lect09_VL3_Simulink/Adaptive Frequency Oscillators ==
  data: theta input; theta_hat output; M input; epsilon input; nu input; dt input; AFO_ON input; state_in input; theta_dot_hat output; theta_ddot_hat output; state_out output
function [theta_hat,theta_dot_hat,theta_ddot_hat, state_out]= AFO(theta,M,epsilon,nu,dt,AFO_ON,state_in)

if AFO_ON == 1

    % I defined state_in as so:
    % [theta_0, omega, phi(1), phi(2), phi(3), phi(4), phi(5), phi(6), a(1), a(2), a(3), a(4), a(5), a(6)]
    % [      1,     2,      3,      4,      5,      6,      7,      8,    9,   10,   11,   12,   13,   14]
    theta_0 = state_in(1);
    omega = state_in(2);
    phi = zeros(M,1);
    for i = 1:M
        phi(i) = state_in(i+2);
    end
    a = zeros(M,1);
    for j = 1:M
        a(j) = state_in(j+8);
    end

    % Error Signal
    sum_a_phi = 0; % the summation at the end of F(t): a_j(t)*sin(phi_j(t)); j = 1,...,M
    for k=1:M
        sum_a_phi = sum_a_phi + a(k)*sin(phi(k));
    end

    F = theta - theta_0 - sum_a_phi;

    % Update Oscillator State
    phi_t_1 = zeros(M,1); % phi(t+1); to pre-allocate memory
    a_t_1 = zeros(M,1); % a(t+1); to pre-allocate memory

    for x = 1:M
        phi_t_1(x) = mod(phi(x) + dt*(x*omega+epsilon*F*cos(phi(x))),2*pi);
        a_t_1(x) = a(x) + dt*(nu*F*sin(phi(x)));
    end

    omega_t_1  = omega + dt*(epsilon*F*cos(phi(1))); % omega_t_1
    theta_0_t_1 = theta_0 + dt*(nu*F); % theta_0(t+1)

    % Update Estimates
    sum_a_phi_t_1 = 0; % summation at the end of theta_hat: a_j(t)*sin(phi_j(t+1)); j = 1,...,M
    for x=1:M
        sum_a_phi_t_1 = sum_a_phi_t_1 + a(x)*sin(phi_t_1(x));
    end

    theta_hat = theta_0_t_1 + sum_a_phi_t_1;

    theta_dot_hat = 0;
    theta_ddot_hat = 0;
    for y = 1:M
        theta_dot_hat = theta_dot_hat + y*omega*a(y)*cos(phi_t_1(y));
        theta_ddot_hat = theta_ddot_hat + y*(omega^2)*a(y)*sin(phi_t_1(y));
    end
    theta_ddot_hat = theta_ddot_hat * -1;
        
    % theta is the signal input; it automatically changes each time step
    % AFO_ON changes automatically each time step
    % state_in needs to be iterated; declaring state_out will automatically become state_in b/c of the feedback
    % the rest of the inputs are constant

    % F(t) is calculated using the other variables each time step

    % Needs to update for next state: a_j, phi_j, omega, theta_0
    omega = omega_t_1;
    theta_0 = theta_0_t_1;
    a = a_t_1;
    phi = phi_t_1;

    state_out = [theta_0, omega, phi(1), phi(2), phi(3), phi(4), phi(5), phi(6), a(1), a(2), a(3), a(4), a(5), a(6)]';

else %If AFO is off.
    theta_hat = 0;
    theta_dot_hat = 0;
    theta_ddot_hat = 0;
    state_out = state_in; %[0, 3*pi/2, pi/2, pi/2, pi/2, pi/2, pi/2, pi/2, 0, 0, 0, 0, 0, 0]'; % state doesn't change until AFO turns on
end

== matlab function ME655_Lect09_VL3_Simulink/CLME ==
  data: big_K input; small_k input; Rhip_p input; Rhip_v input; Rhip_a input; phiP_hat output; phiP_dot_hat output
function [phiP_hat, phiP_dot_hat]= CLME(big_K, small_k, Rhip_p, Rhip_v, Rhip_a)

% healthy states
phiH = [Rhip_p, Rhip_v];
phiH_dot = [Rhip_v, Rhip_a];
phiH_tot = [phiH; phiH_dot];

% Estimated paretic states
% phiP_tot = zeros(2, length(Rhip_p));
% for i = 1:length(Rhip_p)
%     phiP_tot(:,i) = big_K * phiH_tot(i,:)' + small_k;
% end

phiP_tot = big_K * phiH_tot' + small_k;

phiP_hat = phiP_tot(1);
phiP_dot_hat = phiP_tot(2);

== matlab function ME655_Lect09_VL3_Simulink/Kalman Filter ==
  data: x_k_prev input; x_k_next output; P_k_prev input; A input; Q input; R input; H input; Lhip_pos input; P_k_next output; Lhip_pos_des output; Lhip_vel_des output; Lhip_vel input
function [x_k_next, P_k_next, Lhip_pos_des, Lhip_vel_des]= KalmanFilter(x_k_prev, P_k_prev, A, Q, R, H, Lhip_pos, Lhip_vel)

%% Predict

% Project State Ahead
x_k_pred = A * x_k_prev;
% Project Error Covariance Ahead
P_k_pred = A * P_k_prev * A' + Q;

%% Measure

% "Measured" Value from CLME
z = [Lhip_pos; Lhip_vel];

% Kalman Gain
K = P_k_pred * H / (H * P_k_pred * H + R);
% Update Estimate Measurement
x_k_next = x_k_pred + K * (z - H * x_k_pred);
% Update Error Covariance
P_k_next = (eye(2) - K*H)*P_k_pred;

% Output the desired left hip quantities
Lhip_pos_des = x_k_next(1);
Lhip_vel_des = x_k_next(2);

== matlab function ME655_Lect09_VL3_Simulink/RMS1 ==
  data: Act_theta input; RMS_NLF output; RMS_CLME output; Sum_E2_NLF output; Sum_E2_CLME output; Data_points_out output; NLF_theta input; CLME_theta input; Sum_E_NLF input; Sum_E_CLME input; Data_points_in input
function [RMS_NLF, RMS_CLME, Sum_E2_NLF, Sum_E2_CLME, Data_points_out]= fcn(Act_theta, NLF_theta, CLME_theta, Sum_E_NLF, Sum_E_CLME, Data_points_in)

Data_points_out = Data_points_in + 1;
Sum_E2_NLF = Sum_E_NLF + (Act_theta - NLF_theta)^2;
Sum_E2_CLME = Sum_E_CLME + (Act_theta - CLME_theta)^2;
RMS_NLF= (Sum_E2_NLF/Data_points_out)^(0.5);
RMS_CLME= (Sum_E2_CLME/Data_points_out)^(0.5);

== matlab function ME655_Lect09_VL3_Simulink/Tau_InverseDynamic ==
  data: mR input; Tau_tot output; mH input; LR input; LH input; IRC input; IHC input; g input; theta input; theta_dot input; theta_ddot input
function Tau_tot = InverseDynamicModel(mR,mH,LR,LH,IRC,IHC,g,theta,theta_dot,theta_ddot)

% Servo Control
Gain = (IRC + mR*LR^2) + (IHC + mH*LH^2);
% Kh = 9.869604401089358e+02; % taken from Data.mat file
% Bh = 62.831853071795860; % taken from Data.mat file
Human_Controller = theta_ddot; %Kh*theta+Bh*theta_dot+theta_ddot; % Human Controller
Servo_Control = Human_Controller*Gain;

% Gravity Comp Control
TauG_h=mH*g*LH*sin(theta); % human gravity compensation term
TauG_R=mR*g*LR*sin(theta); % robot gravity model
Gravity_Comp_Control = TauG_R + TauG_h;

% Tau_Total
Tau_R = 0;

Tau_H = Servo_Control + Gravity_Comp_Control - Tau_R;

Tau_tot = Tau_H + Tau_R;

== matlab function ME655_Lect09_VL3_Simulink/Tau_InverseDynamic2 ==
  data: mR input; Tau_tot output; mH input; LR input; LH input; IRC input; IHC input; g input; theta input; theta_dot input; theta_ddot input
function Tau_tot = InverseDynamicModel_Q4(mR,mH,LR,LH,IRC,IHC,g,theta,theta_dot,theta_ddot)

% Servo Control
Gain = (IRC + mR*LR^2) + (IHC + mH*LH^2);
% Kh = 9.869604401089358e+02; % taken from Data.mat file
% Bh = 62.831853071795860; % taken from Data.mat file
Human_Controller = theta_ddot; %Kh*theta+Bh*theta_dot+theta_ddot; % Human Controller
Servo_Control = Human_Controller*Gain;

% Gravity Comp Control
TauG_h=mH*g*LH*sin(theta); % human gravity compensation term
TauG_R=mR*g*LR*sin(theta); % robot gravity model
Gravity_Comp_Control = TauG_R + TauG_h;

% Tau_Total
Tau_R = 0;

Tau_H = Servo_Control + Gravity_Comp_Control - Tau_R;

Tau_tot = Tau_H + Tau_R;

== matlab function ME655_Lect09_VL3_Simulink/Leg + Human Control1/human_motor_control/LEG gravity model ==
  data: theta input; mLE input; LLE input; TauG_h output; g input
function TauG_h   = HumanLegGravModel(theta,mLE,LLE,g)
% human gravity compensation term
TauG_h=mLE*g*LLE*sin(theta);

end

== matlab function ME655_Lect09_VL3_Simulink/Leg + Human Control1/human_motor_control/ROBOT gravity model ==
  data: mR input; g input; LR input; theta input; TauG_R output
function TauG_R  = RobotGravModel(mR,g,LR,theta)

TauG_R=mR*g*LR*sin(theta);
% TauG_h=mLE*g*LLE*sin(theta);

end

== matlab function ME655_Lect09_VL3_Simulink/Leg + Human Control1/plant/LEG + ROBOT ==
  data: Tau_h input; Tau_R input; theta input; theta_dd output; IHC input; mH input; LH input; IRC input; mR input; LR input; g input
function theta_dd   = LegRobotModel(Tau_h,Tau_R,theta,IHC,mH,LH,IRC,mR,LR,g)

theta_dd = 1/((IRC + mR*LR^2)+(IHC + mH*LH^2)) * (Tau_h-mH*g*LH*sin(theta) + Tau_R-mR*g*LR*sin(theta));

end
